simulink model "stills_R_W"  (Simulink 7.1)
settings: Solver=FixedStepDiscrete  StartTime=0.0  StopTime=inf  RelTol=1e-3
libraries: rtdxBlocks x2, etargetslib x1, vipconversions x1
settings Model: Creator=greith  LastModifiedBy=karin
settings SolverCC: PositivePriorityOrder=on
settings DataIOCC: SaveOutput=off  SaveTime=off
settings OptimizationCC: OptimizeModelRefInitCode=on
settings DebuggingCC: SaveWithParameterizedLinksMsg=none  SignalResolutionControl=TryResolveAllWithWarning
settings HardwareCC: ProdBitPerLong=40  ProdIntDivRoundTo=Zero  ProdEndianess=LittleEndian  ProdHWDeviceType=Texas Instruments->C6000
settings RTWCC: SystemTargetFile=ccslink_ert.tlc  GenCodeOnly=on  GenerateMakefile=off  TemplateMakefile=ccslink_ert.tmf  Description=Embedded IDE Link CC (ERT) code generation for TMS320(TM) DSP platforms  ProcessScript=ccslink_ert_make_rtw_hook
settings CodeAppCC: IgnoreCustomStorageClasses=off
settings ERTTgtLinkCCS: TargetFcnLib=ansi_tfl_table_tmw.mat  TargetFunctionLibrary=ANSI_C  UtilityFuncGeneration=Auto  GenerateFullHeader=on  GenerateSampleERTMain=off  GenerateTestInterfaces=off  IsPILTarget=off  ModelReferenceCompliant=on  CompOptLevelCompliant=off  IncludeMdlTerminateFcn=on  CombineOutputUpdateFcns=on  SuppressErrorStatus=off  IncludeFileDelimiter=Auto  ERTCustomFileBanners=on  SupportAbsoluteTime=on  LogVarNameModifier=rt_  MatFileLogging=off  MultiInstanceERTCode=off  SupportNonFinite=on  SupportComplex=on  PurelyIntegerCode=off  SupportContinuousTime=off  SupportNonInlinedSFcns=off  EnableShiftOperators=on  ParenthesesLevel=Nominal  PortableWordSizes=off  ModelStepFunctionPrototypeControlCompliant=off  AutosarCompliant=off  GenerateErtSFunction=off  GenerateASAP2=off  ExtMode=off  ExtModeTransport=0  ExtModeStaticAlloc=on  ExtModeStaticAllocSize=1000000  ExtModeTesting=off  ExtModeMexFile=ext_comm  ExtModeIntrfLevel=Level1  InlinedParameterPlacement=NonHierarchical  TargetOS=BareBoardExample  MultiInstanceErrorCode=Error  RateGroupingCode=on  RootIOFormat=Individual arguments  RTWCAPISignals=off  RTWCAPIParams=off  RTWCAPIStates=off  ERTSrcFileBannerTemplate=ert_code_template.cgt  ERTHdrFileBannerTemplate=ert_code_template.cgt  ERTDataSrcFileTemplate=ert_code_template.cgt  ERTDataHdrFileTemplate=ert_code_template.cgt  ERTCustomFileTemplate=example_file_process.tlc  ModuleNamingRule=Unspecified  SignalDisplayLevel=10  ParamTuneLevel=10  GlobalDataDefinition=Auto  DataDefinitionFile=global.c  GlobalDataReference=Auto  DataReferenceFile=global.h  GRTInterface=off  PreserveExpressionOrder=off  PreserveIfCondition=off  EnableUserReplacementTypes=off  MemSecPackage=--- None ---  MemSecDataConstants=Default  MemSecDataIO=Default  MemSecDataInternal=Default  MemSecDataParameters=Default  MemSecFuncInitTerm=Default  MemSecFuncExecute=Default  exportIDEObj=on  ideObjName=CCS_Obj  oldideObjName=CCS_Obj  ideObjTimeout=10  oldideObjTimeout=10  ideObjBuildTimeout=1000  oldideObjBuildTimeout=1000  ProfileGenCode=off  ProfileNumSamples=100  InlineDSPBlks=on  projectOptions=Custom  debugCompilerOptions="-g -d\"_DEBUG\""  releaseCompilerOptions=-o2  getCompilerOptions=off  getLinkerOptions=off  systemStackSize=8192  buildAction=Build_and_execute  overrunNotificationMethod=None  overrunNotificationFcn=myfunction  oldoverrunNotificationFcn=myfunction  configurePIL=off  configPILBlockAction=Create_PIL_block_build_and_download

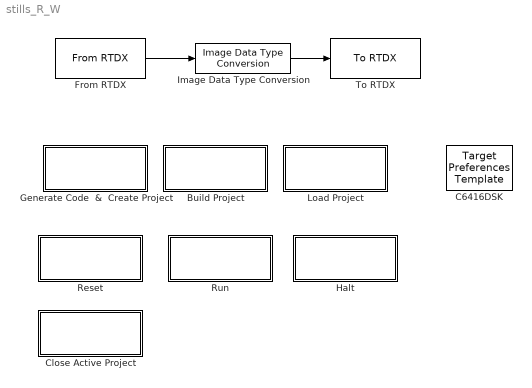
== system stills_R_W ==
  Build Project : Subsystem
      settings: OpenFcn=CCS_Obj.build;
      mask Display: disp('Build\nProject')
  C6416DSK : etargetslib/Target Preferences Template  Tag=ccslinktgtpref  SystemSampleTime=-1
  Close Active Project : Subsystem
      settings: OpenFcn=close(CCS_Obj,[],'project')
      mask Display: disp('Close Active Project')
  From RTDX : rtdxBlocks/From RTDX  channelNameStr=inputimage  isBlocking=on  icMaskVar=0  Ts=-1  dims=[65 309]  isFrame=off  dType=uint8  isChannelEnabled=on  isHighSpeedRTDXUsed=on
  Generate Code  &  Create Project : Subsystem
      settings: OpenFcn=make_rtw;
      mask Display: disp('Generate Code\n & \nCreate Project')
  Halt : Subsystem
      settings: OpenFcn=CCS_Obj.halt;
      mask Display: disp('Halt')
  Image Data Type Conversion : vipconversions/Image Data Type Conversion  outDT=uint8  isSigned=on  wordLen=16  numFracBits=0
  Load Project : Subsystem
      settings: OpenFcn=CCS_Obj.load([pwd,'\',bdroot,'_c6000_rtw\', bdroot, '.out'])
      mask Display: disp('Load\nProject')
  Reset : Subsystem
      settings: OpenFcn=CCS_Obj.reset;
      mask Display: disp('Reset')
  Run : Subsystem
      settings: OpenFcn=CCS_Obj.run;
      mask Display: disp('Run')
  To RTDX : rtdxBlocks/To RTDX  channelNameStr=outputimage  isBlocking=on  isChannelEnabled=on
  wires:
  From RTDX/1 -> Image Data Type Conversion/1
  Image Data Type Conversion/1 -> To RTDX/1

== system stills_R_W/Build Project ==

== system stills_R_W/Close Active Project ==

== system stills_R_W/Generate Code  &  Create Project ==

== system stills_R_W/Halt ==

== system stills_R_W/Load Project ==

== system stills_R_W/Reset ==

== system stills_R_W/Run ==
